simulink model "malt_test_angle"  (R2023a)
settings: Solver=FixedStepAuto  StartTime=0.0  StopTime=50  FixedStep=framePeriod_s  RelTol=1e-3
undefined symbols (not defined in the file or in its folder): Aircraft, DiscIntNeverNeededParam, framePeriod_s, frameRate_hz
libraries: simulink x29, slpidlib x8, simulink_extras x3
(part 1 of 2)
settings Model: Creator=brian  LastModifiedBy=tuan
settings SolverCC: AlgebraicLoopSolver=TrustRegion
settings OptimizationCC: DefaultParameterBehavior=Inlined  GainParamInheritBuiltInType=on  UseFloatMulNetSlope=on  DefaultUnderspecifiedDataType=single  InlineInvariantSignals=on  OptimizeBlockIOStorage=off  PassReuseOutputArgsAs=Individual arguments  ZeroExternalMemoryAtStartup=off  ZeroInternalMemoryAtStartup=off  NoFixptDivByZeroProtection=on  EfficientFloat2IntCast=on  LifeSpan=1  OptimizeBlockOrder=speed  DifferentSizesBufferReuse=on  EfficientTunableParamExpr=on
settings DebuggingCC: ParameterTunabilityLossMsg=error  UnconnectedInputMsg=warning  UnconnectedOutputMsg=warning  UnconnectedLineMsg=warning
settings HardwareCC: ProdBitPerPointer=32  ProdBitPerSizeT=32  ProdBitPerPtrDiffT=32  ProdLargestAtomicInteger=Long  ProdLargestAtomicFloat=Double  ProdWordSize=32  ProdLongLongMode=on  ProdHWDeviceType=NXP->Cortex-M4
settings ModelReferenceCC: EnableRefExpFcnMdlSchedulingChecks=on  ModelReferenceNumInstancesAllowed=Single
settings SFSimCC: SimParseCustomCode=off  MATLABDynamicMemAlloc=off  SimTargetLang=C++
settings RTWCC: Description=Embedded Coder  SystemTargetFile=ert.tlc  GenCodeOnly=on  TemplateMakefile=ert_default_tmf  GenerateReport=on  RTWVerbose=off  Toolchain=GNU gcc/g++ | gmake (64-bit Linux)  BuildConfiguration=Faster Runs  IncludeHyperlinkInReport=on  TargetLang=C++  GenerateTraceInfo=on  DLArmComputeVersion=19.05
settings CodeAppCC: ForceParamTrailComments=on  IgnoreCustomStorageClasses=off  OperatorAnnotations=on  SimulinkDataObjDesc=on  SFDataObjDesc=on  CustomSymbolStrGlobalVar=rt$N$M  CustomSymbolStrType=$N$M  CustomSymbolStrFcn=$N$M$F  CustomSymbolStrMacro=$N$M  InsertBlockDesc=on
settings ERTTargetCC: TargetLangStandard=C++11 (ISO)  IncludeMdlTerminateFcn=off  CombineSignalStateStructs=on  SuppressErrorStatus=on  SupportAbsoluteTime=off  CodeInterfacePackaging=C++ class  SupportComplex=off  ERTHeaderFileRootName=autocode$E  ERTSourceFileRootName=autocode$E  InlinedParameterPlacement=NonHierarchical  RootIOFormat=Structure reference  ERTCustomFileTemplate=example_file_process.tlc  ERTFilePackagingFormat=Compact  ArrayContainerType=std::array

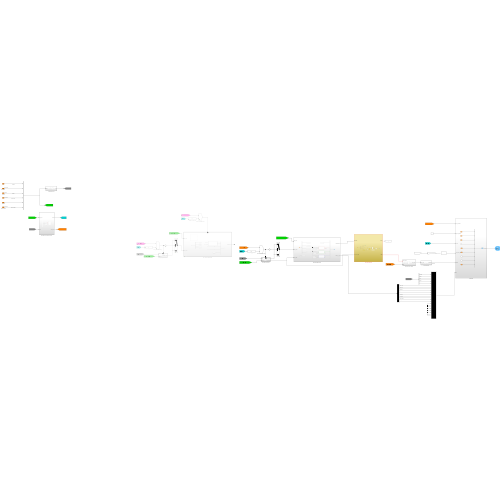
[thumbnail: Simulink's stored preview of the top-level diagram]
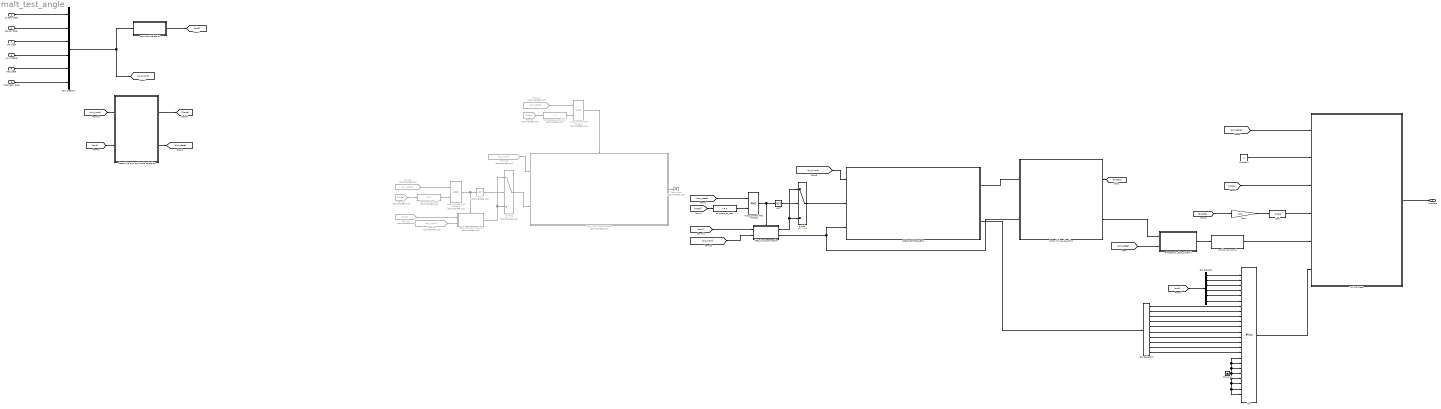
== system malt_test_angle ==
  System Data : Inport  OutDataTypeStr=Bus: SysData  SampleTime=framePeriod_s  BusOutputAsStruct=on
  Sensor Data : Inport  Port=2  OutDataTypeStr=Bus: SensorData  SampleTime=framePeriod_s  BusOutputAsStruct=on
  INS Data : Inport  Port=3  OutDataTypeStr=Bus: InsData  SampleTime=framePeriod_s  BusOutputAsStruct=on
  AuxInsData : Inport  Port=4  OutDataTypeStr=Bus: AuxInsData  SampleTime=framePeriod_s  BusOutputAsStruct=on
  ADC Data : Inport  Port=5  OutDataTypeStr=Bus: AdcData  SampleTime=framePeriod_s  BusOutputAsStruct=on
  Telemetry Data : Inport  Port=6  OutDataTypeStr=Bus: TelemData  SampleTime=framePeriod_s  BusOutputAsStruct=on
  ANGLE CONTROLLER1 : Subsystem
  Bus Creator1 : BusCreator  Inputs=6
  Bus Selector : BusSelector  OutputSignals=throttle,pitch,roll,yaw,e_stop,mode
  Bus Selector1 : BusSelector  OutputSignals=rate_cmd,rate error,signal3,signal4,signal5,D control,control cc,angle_cmd,pitch_rad,angle_e
  Cast : DataTypeConversion  OutDataTypeStr=single  SaturateOnIntegerOverflow=off  RndMeth=Floor
  Constant : Constant  Value=0  OutDataTypeStr=boolean
  From13 : From  Commented=on  GotoTag=cmd
  From15 : From  Commented=on  GotoTag=arm_state
  From16 : From  Commented=on  GotoTag=Mode
  From18 : From  Commented=on  GotoTag=sys_input
  From19 : From  Commented=on  GotoTag=sys_input
  From20 : From  Commented=on  GotoTag=arm_state
  From21 : From  Commented=on  GotoTag=Mode
  Gain : Gain  Gain=100
  Ground1 : Ground
  Motor Mixing Algorithm : Subsystem
  Mux : Mux  Inputs=24
  NOT : Logic  Operator=NOT  IconShape=distinctive  AllPortsSameDT=off  OutDataTypeStr=boolean
  NOT1 : Logic  Commented=on  Operator=NOT  IconShape=distinctive  AllPortsSameDT=off  OutDataTypeStr=boolean
  POS_HOLD CONTROLLER : Subsystem  Commented=on
  Stab_input_conversion : Subsystem
  Stab_input_conversion1 : Subsystem  Commented=on
  Switch : Switch  Criteria=u2 > Threshold  Threshold=0.5  SaturateOnIntegerOverflow=off  InputSameDT=off
  Switch1 : Switch  Commented=on  Criteria=u2 > Threshold  Threshold=0.5  SaturateOnIntegerOverflow=off  InputSameDT=off
  Terminator : Terminator  Commented=on
  To VMS Data : Subsystem
  cmd to raw pwm1 : Subsystem
  command selection : Subsystem
  compare_to_pos_hold : simulink/Logic and Bit Operations/Compare To Constant  Commented=on  relop=>  const=0  OutDataTypeStr=boolean
  compare_to_stab : simulink/Logic and Bit Operations/Compare To Constant  relop=>=  const=0  OutDataTypeStr=boolean
  compare_to_stab1 : simulink/Logic and Bit Operations/Compare To Constant  Commented=on  relop===  const=1  OutDataTypeStr=boolean
  determine arm and mode selection : Subsystem
  emergency_stop_system1 : Subsystem
  motor_armed AND mode_0 : Logic  IconShape=distinctive  AllPortsSameDT=off  OutDataTypeStr=boolean
  motor_armed AND mode_1 : Logic  Commented=on  IconShape=distinctive  AllPortsSameDT=off  OutDataTypeStr=boolean
  motor_armed AND mode_5 : Logic  Commented=on  IconShape=distinctive  AllPortsSameDT=off  OutDataTypeStr=boolean
  VmsData : Outport  OutDataTypeStr=Bus: VmsData  SampleTime=framePeriod_s  BusOutputAsStruct=on
  wires:
  To VMS Data/1(VmsData) -> VmsData/1  "VmsData"
  [Mode] -> To VMS Data/3(Mode in)
  Constant/1 -> To VMS Data/2(waypoint_reached)
  [arm_state] -> To VMS Data/1(motors_enabled)
  Cast/1 -> To VMS Data/4(throttle_cmd_prcnt)
  [throttle] -> Gain/1
  Gain/1 -> Cast/1
  determine arm and mode selection/2(arm_state) -> [arm_state]
  command selection/1(cmd) -> [cmd]
  determine arm and mode selection/1(mode) -> [Mode]
  Bus Creator1/1 -> command selection/1(InBus), [sys_input]
  [cmd] -> determine arm and mode selection/2(Cmd)
  [sys_input] -> determine arm and mode selection/1(sys_input)
  Motor Mixing Algorithm/2(PWM) -> emergency_stop_system1/1(input_signal)
  cmd to raw pwm1/1(PwmCmd) -> To VMS Data/5(PWM In)  "PwmCmd"
  emergency_stop_system1/1(pwm_cmd) -> cmd to raw pwm1/1(pwm_cmd)
  Mux/1 -> To VMS Data/6(Aux)
  [cmd] -> Bus Selector/1
  Bus Selector/1 -> Mux/1  "<throttle>"
  Bus Selector/2 -> Mux/2  "<pitch>"
  Bus Selector/3 -> Mux/3  "<roll>"
  Bus Selector/4 -> Mux/4  "<yaw>"
  Bus Selector/5 -> Mux/5  "<e_stop>"
  Bus Selector/6 -> Mux/6  "<mode>"
  [arm_state] -> emergency_stop_system1/2(arm)
  Motor Mixing Algorithm/1(throttle) -> [throttle]
  compare_to_stab/1 -> motor_armed AND mode_0/2
  [cmd] -> Stab_input_conversion/1(cmd)
  [sys_input] -> ANGLE CONTROLLER1/1(Sys_input)
  NOT/1 -> Switch/2
  [arm_state] -> motor_armed AND mode_0/1
  motor_armed AND mode_0/1 -> Stab_input_conversion/Enable, NOT/1
  Stab_input_conversion/1(angle_ctrl_input) -> Switch/3, Switch/1
  Switch/1 -> ANGLE CONTROLLER1/2(Cmd_input)
  [Mode] -> compare_to_stab/1
  ANGLE CONTROLLER1/1(Command out) -> Motor Mixing Algorithm/1(MMA Bus)
  ANGLE CONTROLLER1/2(inner_loop_log) -> Bus Selector1/1
  compare_to_pos_hold/1 -> motor_armed AND mode_1/2
  motor_armed AND mode_5/1 -> Stab_input_conversion1/Enable, NOT1/1
  From13/1 -> Stab_input_conversion1/1(cmd)
  From16/1 -> compare_to_pos_hold/1
  From15/1 -> motor_armed AND mode_1/1
  Switch1/1 -> POS_HOLD CONTROLLER/2(Cmd_input)
  NOT1/1 -> Switch1/2
  Stab_input_conversion1/1(angle_ctrl_input) -> Switch1/1, Switch1/3
  From20/1 -> motor_armed AND mode_5/1
  From19/1 -> POS_HOLD CONTROLLER/1(Sys_input)
  From21/1 -> compare_to_stab1/1
  motor_armed AND mode_1/1 -> POS_HOLD CONTROLLER/Enable
  compare_to_stab1/1 -> motor_armed AND mode_5/2
  [sys_input] -> Stab_input_conversion/2(sys input)
  Ground1/1 -> Mux/19, Mux/18, Mux/17, Mux/21, Mux/22, Mux/23, Mux/24, Mux/20
  From18/1 -> Stab_input_conversion1/2(sys input)
  Stab_input_conversion/2(low_throttle) -> ANGLE CONTROLLER1/3(low_thottle), Motor Mixing Algorithm/2(low_throttle_flag)
  System Data/1 -> Bus Creator1/1  "Sys Data"
  AuxInsData/1 -> Bus Creator1/4  "Aux Ins Data"
  Telemetry Data/1 -> Bus Creator1/6  "Telemetry Data"
  Sensor Data/1 -> Bus Creator1/2  "Sensor Data"
  INS Data/1 -> Bus Creator1/3  "Ins Data"
  ADC Data/1 -> Bus Creator1/5  "ADC Data"
  POS_HOLD CONTROLLER/1(Command out) -> Terminator/1
  Bus Selector1/2 -> Mux/8  "<rate error>"
  Bus Selector1/3 -> Mux/9  "<signal3>"
  Bus Selector1/4 -> Mux/10  "<signal4>"
  Bus Selector1/5 -> Mux/11  "<signal5>"
  Bus Selector1/6 -> Mux/12  "<D control>"
  Bus Selector1/7 -> Mux/13  "<control cc>"
  Bus Selector1/1 -> Mux/7  "<rate_cmd>"
  Bus Selector1/8 -> Mux/14  "<angle_cmd>"
  Bus Selector1/9 -> Mux/15  "<pitch_rad>"
  Bus Selector1/10 -> Mux/16  "<angle_e>"

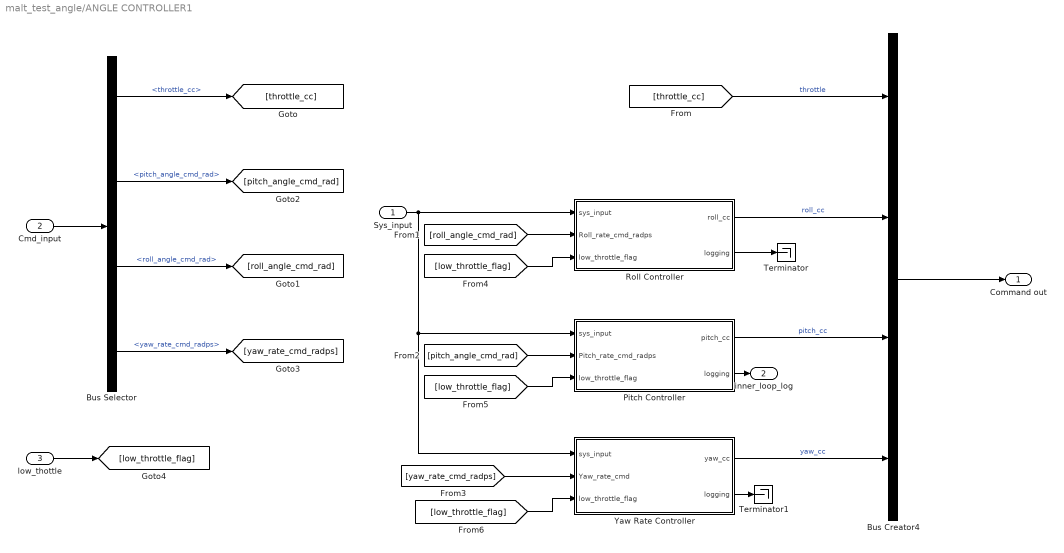
== system malt_test_angle/ANGLE CONTROLLER1 ==
  Sys_input : Inport
  Cmd_input : Inport  Port=2
  low_thottle : Inport  Port=3
  Bus Creator4 : BusCreator  Inputs=4
  Bus Selector : BusSelector  OutputSignals=throttle_cc,pitch_angle_cmd_rad,roll_angle_cmd_rad,yaw_rate_cmd_radps
  Pitch Controller : Subsystem
  Roll Controller : Subsystem
  Terminator : Terminator
  Terminator1 : Terminator
  Yaw Rate Controller : Subsystem
  Command out : Outport
  inner_loop_log : Outport  Port=2
  wires:
  Bus Creator4/1 -> Command out/1
  Cmd_input/1 -> Bus Selector/1
  Yaw Rate Controller/1(yaw_cc) -> Bus Creator4/4  "yaw_cc"
  Pitch Controller/1(pitch_cc) -> Bus Creator4/3  "pitch_cc"
  Roll Controller/1(roll_cc) -> Bus Creator4/2  "roll_cc"
  Sys_input/1 -> Yaw Rate Controller/1(sys_input), Pitch Controller/1(sys_input), Roll Controller/1(sys_input)
  Bus Selector/1 -> [throttle_cc]  "<throttle_cc>"
  Bus Selector/4 -> [yaw_rate_cmd_radps]  "<yaw_rate_cmd_radps>"
  Bus Selector/2 -> [pitch_angle_cmd_rad]  "<pitch_angle_cmd_rad>"
  Bus Selector/3 -> [roll_angle_cmd_rad]  "<roll_angle_cmd_rad>"
  [throttle_cc] -> Bus Creator4/1  "throttle"
  [roll_angle_cmd_rad] -> Roll Controller/2(Roll_rate_cmd_radps)
  [pitch_angle_cmd_rad] -> Pitch Controller/2(Pitch_rate_cmd_radps)
  [yaw_rate_cmd_radps] -> Yaw Rate Controller/2(Yaw_rate_cmd)
  low_thottle/1 -> [low_throttle_flag]
  [low_throttle_flag] -> Roll Controller/3(low_throttle_flag)
  [low_throttle_flag] -> Pitch Controller/3(low_throttle_flag)
  [low_throttle_flag] -> Yaw Rate Controller/3(low_throttle_flag)
  Roll Controller/2(logging) -> Terminator/1
  Yaw Rate Controller/2(logging) -> Terminator1/1
  Pitch Controller/2(logging) -> inner_loop_log/1

== system malt_test_angle/Motor Mixing Algorithm ==
  MMA Bus : Inport
  low_throttle_flag : Inport  Port=2
  Bus Selector : BusSelector  OutputSignals=throttle,roll_cc,pitch_cc,yaw_cc
  Constant : Constant
  Constant1 : Constant  Value=Aircraft.Control.motor_spin_min
  Constant2 : Constant  Value=[0 0 0 0 0 0 0 0]
  Motor Mix : Constant  Value=Aircraft.Motor.mix  OutDataTypeStr=single
  Multiply : Product  Inputs=**  Multiplication=Matrix(*)  OutDataTypeStr=single
  Mux : Mux
  Reshape : Reshape  OutputDimensionality=Row vector (2-D)
  Saturation Dynamic : simulink/Discontinuities/Saturation Dynamic  OutMin=[]  OutMax=[]  OutDataTypeStr=Inherit: Same as second input  OutDataType=fixdt(1, 16)  OutScaling=2^-10  DoSatur=off
  Switch : Switch  Criteria=u2 > Threshold  SaturateOnIntegerOverflow=off  InputSameDT=off
  Transpose : Math  Operator=transpose
  throttle : Outport
  PWM : Outport  Port=2
  wires:
  Mux/1 -> Reshape/1
  Reshape/1 -> Multiply/1
  Motor Mix/1 -> Transpose/1
  MMA Bus/1 -> Bus Selector/1
  Bus Selector/1 -> throttle/1, Mux/1  "<throttle>"
  Transpose/1 -> Multiply/2
  Saturation Dynamic/1 -> PWM/1
  Constant/1 -> Saturation Dynamic/1
  Constant1/1 -> Saturation Dynamic/3
  Bus Selector/2 -> Mux/2  "<roll_cc>"
  Bus Selector/3 -> Mux/3  "<pitch_cc>"
  Bus Selector/4 -> Mux/4  "<yaw_cc>"
  Switch/1 -> Saturation Dynamic/2
  low_throttle_flag/1 -> Switch/2
  Multiply/1 -> Switch/3  "Command"
  Constant2/1 -> Switch/1

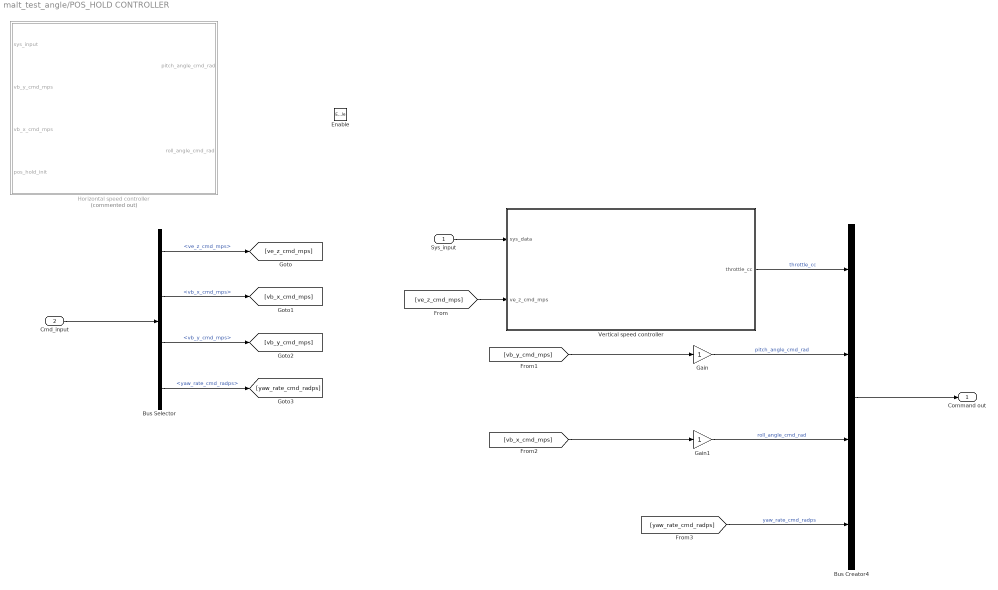
== system malt_test_angle/POS_HOLD CONTROLLER ==
  Sys_input : Inport
  Cmd_input : Inport  Port=2
  Enable : EnablePort  StatesWhenEnabling=reset  PropagateVarSize=During execution
  Bus Creator4 : BusCreator  Inputs=4
  Bus Selector : BusSelector  OutputSignals=ve_z_cmd_mps,vb_x_cmd_mps,vb_y_cmd_mps,yaw_rate_cmd_radps
  Gain : Gain
  Gain1 : Gain
  Horizontal speed controller : Subsystem  Commented=on
  Vertical speed controller : Subsystem
  Command out : Outport
  wires:
  Bus Creator4/1 -> Command out/1
  Bus Selector/1 -> [ve_z_cmd_mps]  "<ve_z_cmd_mps>"
  Bus Selector/2 -> [vb_x_cmd_mps]  "<vb_x_cmd_mps>"
  Bus Selector/3 -> [vb_y_cmd_mps]  "<vb_y_cmd_mps>"
  Bus Selector/4 -> [yaw_rate_cmd_radps]  "<yaw_rate_cmd_radps>"
  [yaw_rate_cmd_radps] -> Bus Creator4/4  "yaw_rate_cmd_radps"
  Cmd_input/1 -> Bus Selector/1
  Vertical speed controller/1(throttle_cc) -> Bus Creator4/1  "throttle_cc"
  [vb_y_cmd_mps] -> Gain/1
  [vb_x_cmd_mps] -> Gain1/1
  Sys_input/1 -> Vertical speed controller/1(sys_data)
  [ve_z_cmd_mps] -> Vertical speed controller/2(ve_z_cmd_mps)
  Gain/1 -> Bus Creator4/2  "pitch_angle_cmd_rad"
  Gain1/1 -> Bus Creator4/3  "roll_angle_cmd_rad"

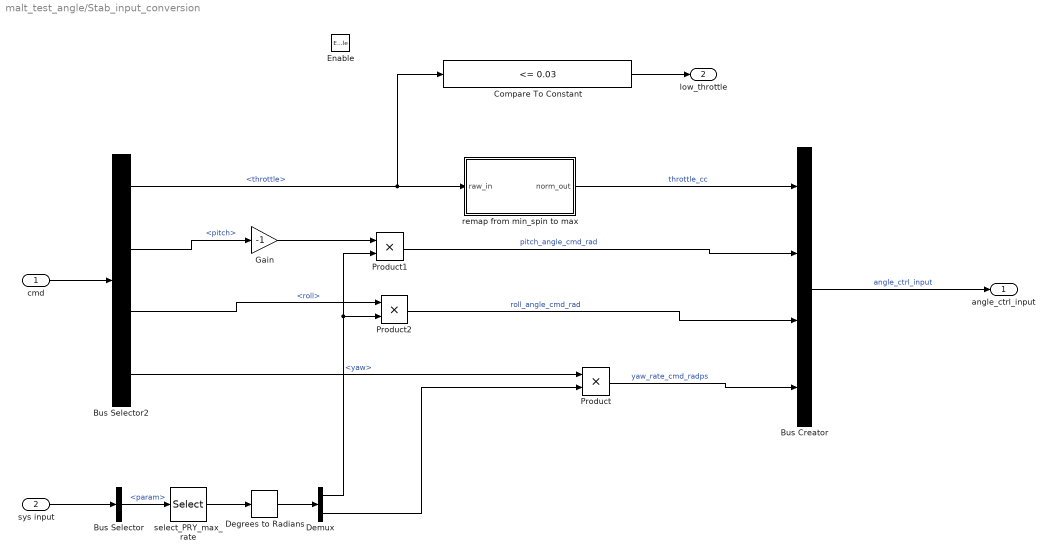
== system malt_test_angle/Stab_input_conversion ==
  cmd : Inport
  sys input : Inport  Port=2
  Enable : EnablePort
  Bus Creator : BusCreator  Inputs=4
  Bus Selector : BusSelector  OutputSignals=Telemetry Data.param
  Bus Selector2 : BusSelector  OutputSignals=throttle,pitch,roll,yaw
  Compare To Constant : simulink/Logic and Bit Operations/Compare To Constant  relop=<=  const=0.03  OutDataTypeStr=boolean
  Degrees to Radians : simulink_extras/Transformations/Degrees to Radians
  Demux : Demux  Outputs=2
  Gain : Gain  Gain=-1
  Product : Product
  Product1 : Product
  Product2 : Product
  remap from min_spin to max : Subsystem
  select_PRY_max_rate : Selector  IndexMode=Zero-based  IndexOptions=Index vector (dialog)  Indices=[13 12]  OutputSizes=1
  angle_ctrl_input : Outport
  low_throttle : Outport  Port=2
  wires:
  Bus Selector2/3 -> Product2/1  "<roll>"
  Product2/1 -> Bus Creator/3  "roll_angle_cmd_rad"
  Bus Selector2/2 -> Gain/1  "<pitch>"
  Bus Creator/1 -> angle_ctrl_input/1  "angle_ctrl_input"
  Product1/1 -> Bus Creator/2  "pitch_angle_cmd_rad"
  cmd/1 -> Bus Selector2/1
  Bus Selector2/1 -> Compare To Constant/1, remap from min_spin to max/1(raw_in)  "<throttle>"
  Product/1 -> Bus Creator/4  "yaw_rate_cmd_radps"
  Bus Selector2/4 -> Product/1  "<yaw>"
  remap from min_spin to max/1(norm_out) -> Bus Creator/1  "throttle_cc"
  Compare To Constant/1 -> low_throttle/1
  sys input/1 -> Bus Selector/1
  Bus Selector/1 -> select_PRY_max_rate/1  "<param>"
  select_PRY_max_rate/1 -> Degrees to Radians/1
  Demux/2 -> Product/2
  Gain/1 -> Product1/1
  Demux/1 -> Product2/2, Product1/2
  Degrees to Radians/1 -> Demux/1

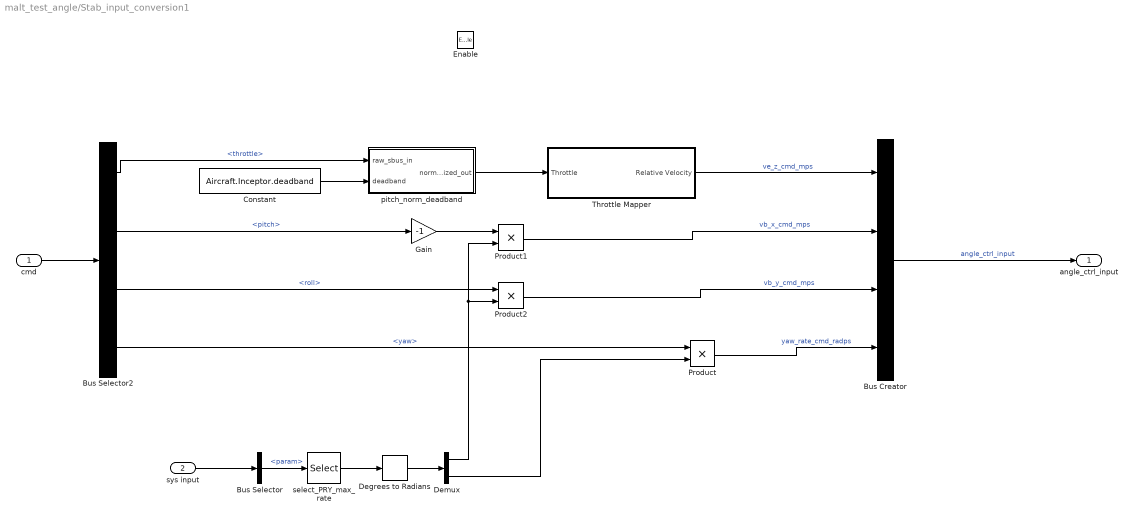
== system malt_test_angle/Stab_input_conversion1 ==
  cmd : Inport
  sys input : Inport  Port=2
  Enable : EnablePort
  Bus Creator : BusCreator  Inputs=4
  Bus Selector : BusSelector  OutputSignals=Telemetry Data.param
  Bus Selector2 : BusSelector  OutputSignals=throttle,pitch,roll,yaw
  Constant : Constant  Value=Aircraft.Inceptor.deadband
  Degrees to Radians : simulink_extras/Transformations/Degrees to Radians
  Demux : Demux  Outputs=2
  Gain : Gain  Gain=-1
  Product : Product
  Product1 : Product
  Product2 : Product
  Throttle Mapper : Subsystem
  pitch_norm_deadband : Subsystem
  select_PRY_max_rate : Selector  IndexMode=Zero-based  IndexOptions=Index vector (dialog)  Indices=[13 12]  OutputSizes=1
  angle_ctrl_input : Outport
  wires:
  Bus Selector2/3 -> Product2/1  "<roll>"
  Product2/1 -> Bus Creator/3  "vb_y_cmd_mps"
  Bus Selector2/2 -> Gain/1  "<pitch>"
  Bus Creator/1 -> angle_ctrl_input/1  "angle_ctrl_input"
  Product1/1 -> Bus Creator/2  "vb_x_cmd_mps"
  cmd/1 -> Bus Selector2/1
  Product/1 -> Bus Creator/4  "yaw_rate_cmd_radps"
  Bus Selector2/4 -> Product/1  "<yaw>"
  Throttle Mapper/1(Relative Velocity) -> Bus Creator/1  "ve_z_cmd_mps"
  sys input/1 -> Bus Selector/1
  Bus Selector/1 -> select_PRY_max_rate/1  "<param>"
  select_PRY_max_rate/1 -> Degrees to Radians/1
  Demux/2 -> Product/2
  Gain/1 -> Product1/1
  Demux/1 -> Product2/2, Product1/2
  Degrees to Radians/1 -> Demux/1
  Bus Selector2/1 -> pitch_norm_deadband/1(raw_sbus_in)  "<throttle>"
  pitch_norm_deadband/1(normalized_out) -> Throttle Mapper/1(Throttle)
  Constant/1 -> pitch_norm_deadband/2(deadband)

== system malt_test_angle/To VMS Data ==
  motors_enabled : Inport
  waypoint_reached : Inport  Port=2
  Mode in : Inport  Port=3
  throttle_cmd_prcnt : Inport  Port=4
  PWM In : Inport  Port=5
  Aux : Inport  Port=6
  Bus Creator : BusCreator  Inputs=9  OutDataTypeStr=Bus: VmsData  NonVirtualBus=on
      settings: InheritFromInputs=off
  Ground : Ground
  Ground1 : Ground
  Ground2 : Ground
  VmsData : Outport
  wires:
  Bus Creator/1 -> VmsData/1
  waypoint_reached/1 -> Bus Creator/1  "advance_waypoint"
  motors_enabled/1 -> Bus Creator/2  "motors_enabled"
  Mode in/1 -> Bus Creator/3  "mode"
  Ground1/1 -> Bus Creator/4  "sbus"
  PWM In/1 -> Bus Creator/5  "pwm"
  throttle_cmd_prcnt/1 -> Bus Creator/6  "throttle_cmd_prcnt"
  Aux/1 -> Bus Creator/9  "aux"
  Ground/1 -> Bus Creator/7  "flight_time_remaining_s"
  Ground2/1 -> Bus Creator/8  "power_remaining_prcnt"

== system malt_test_angle/cmd to raw pwm1 ==
  note: cnt - pwm output to actual hardware
  pwm_cmd : Inport
  Data Type Conversion : DataTypeConversion  OutDataTypeStr=int16  SaturateOnIntegerOverflow=off  RndMeth=Floor
  motor_PWM_denormalize : Subsystem
  PwmCmd : Outport
  wires:
  pwm_cmd/1 -> motor_PWM_denormalize/1(normalized_input)  "cmd"
  motor_PWM_denormalize/1(raw_output) -> Data Type Conversion/1
  Data Type Conversion/1 -> PwmCmd/1  "cnt"

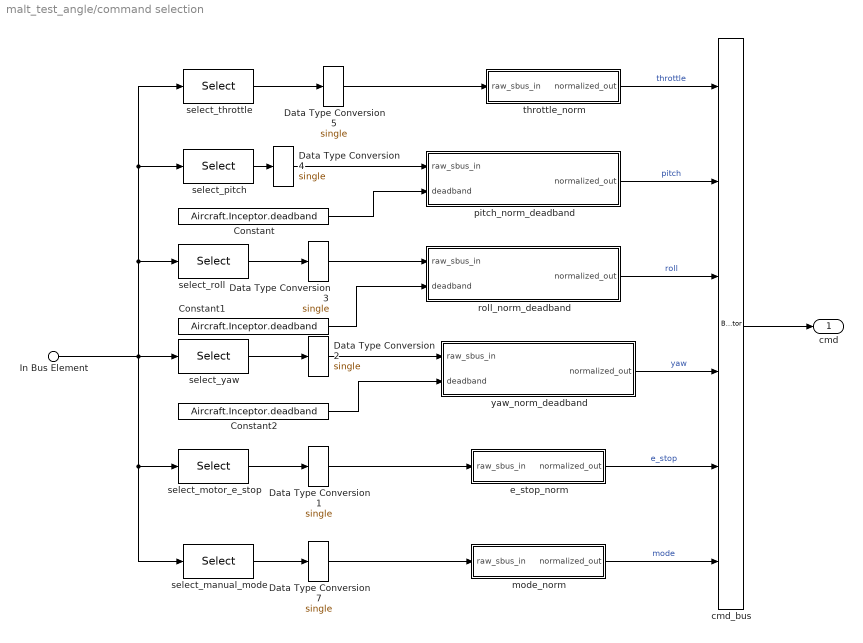
== system malt_test_angle/command selection ==
  In Bus Element : Inport  PortName=InBus  Element=Sensor Data.inceptor.ch
  Constant : Constant  Value=Aircraft.Inceptor.deadband
  Constant1 : Constant  Value=Aircraft.Inceptor.deadband
  Constant2 : Constant  Value=Aircraft.Inceptor.deadband
  Data Type Conversion{1..5,7} (6 alike) : DataTypeConversion  OutDataTypeStr=single  SaturateOnIntegerOverflow=off  RndMeth=Floor
  cmd_bus : BusCreator  Inputs=6
  e_stop_norm : Subsystem
  mode_norm : Subsystem
  pitch_norm_deadband : Subsystem
  roll_norm_deadband : Subsystem
  select_manual_mode : Selector  IndexOptions=Index vector (dialog)  Indices=Aircraft.Inceptor.mode0  OutputSizes=1
  select_motor_e_stop : Selector  IndexOptions=Index vector (dialog)  Indices=Aircraft.Inceptor.throttle_e_stop  OutputSizes=1
  select_pitch : Selector  IndexOptions=Index vector (dialog)  Indices=Aircraft.Inceptor.pitch  OutputSizes=1
  select_roll : Selector  IndexOptions=Index vector (dialog)  Indices=Aircraft.Inceptor.roll  OutputSizes=1
  select_throttle : Selector  IndexOptions=Index vector (dialog)  Indices=Aircraft.Inceptor.throttle  OutputSizes=1
  select_yaw : Selector  IndexOptions=Index vector (dialog)  Indices=Aircraft.Inceptor.yaw  OutputSizes=1
  throttle_norm : Subsystem
  yaw_norm_deadband : Subsystem
  cmd : Outport
  wires:
  select_pitch/1 -> Data Type Conversion4/1
  select_yaw/1 -> Data Type Conversion2/1
  select_throttle/1 -> Data Type Conversion5/1
  cmd_bus/1 -> cmd/1
  Data Type Conversion5/1 -> throttle_norm/1(raw_sbus_in)
  select_roll/1 -> Data Type Conversion3/1
  In Bus Element/1 -> select_roll/1, select_throttle/1, select_pitch/1, select_manual_mode/1, select_motor_e_stop/1, select_yaw/1
  Data Type Conversion1/1 -> e_stop_norm/1(raw_sbus_in)
  select_motor_e_stop/1 -> Data Type Conversion1/1
  Data Type Conversion7/1 -> mode_norm/1(raw_sbus_in)
  select_manual_mode/1 -> Data Type Conversion7/1
  Data Type Conversion2/1 -> yaw_norm_deadband/1(raw_sbus_in)
  Constant2/1 -> yaw_norm_deadband/2(deadband)
  throttle_norm/1(normalized_out) -> cmd_bus/1  "throttle"
  roll_norm_deadband/1(normalized_out) -> cmd_bus/3  "roll"
  pitch_norm_deadband/1(normalized_out) -> cmd_bus/2  "pitch"
  Data Type Conversion4/1 -> pitch_norm_deadband/1(raw_sbus_in)
  Constant/1 -> pitch_norm_deadband/2(deadband)
  Constant1/1 -> roll_norm_deadband/2(deadband)
  Data Type Conversion3/1 -> roll_norm_deadband/1(raw_sbus_in)
  yaw_norm_deadband/1(normalized_out) -> cmd_bus/4  "yaw"
  e_stop_norm/1(normalized_out) -> cmd_bus/5  "e_stop"
  mode_norm/1(normalized_out) -> cmd_bus/6  "mode"

== system malt_test_angle/determine arm and mode selection ==
  sys_input : Inport
  Cmd : Inport  Port=2
  Bus Selector : BusSelector  OutputSignals=Sensor Data.inceptor,Ins Data.initialized
  Bus Selector1 : BusSelector  OutputSignals=e_stop,mode,yaw,throttle
  Failsafe_management : Subsystem
  OR1 : Logic  Operator=OR  IconShape=distinctive  AllPortsSameDT=off  OutDataTypeStr=boolean
  Subsystem : Subsystem
  mode_type_conversion : DataTypeConversion  OutDataTypeStr=int8  RndMeth=Nearest  SaturateOnIntegerOverflow=off
  nav_init AND motor_enable : Logic  IconShape=distinctive  AllPortsSameDT=off  OutDataTypeStr=boolean
  yaw_stick_arming : Subsystem
  mode : Outport
  arm_state : Outport  Port=2
  wires:
  Failsafe_management/1(radio_failsafe_enabled) -> [radio_failsafe_enabled]
  nav_init AND motor_enable/1 -> arm_state/1, Failsafe_management/3(motor_state)
  Bus Selector/2 -> nav_init AND motor_enable/2  "<initialized>"
  sys_input/1 -> Bus Selector/1
  [motor_e_stop] -> yaw_stick_arming/3(e_stop)
  Bus Selector1/4 -> yaw_stick_arming/2(<throttle>)  "<throttle>"
  Bus Selector1/2 -> mode_type_conversion/1  "<mode>"
  Bus Selector1/3 -> yaw_stick_arming/1(<yaw>)  "<yaw>"
  Bus Selector1/1 -> Subsystem/1(<e_stop>)  "<e_stop>"
  mode_type_conversion/1 -> mode/1, Failsafe_management/2(manual_mode)
  Cmd/1 -> Bus Selector1/1
  yaw_stick_arming/1(arm_state) -> nav_init AND motor_enable/1
  OR1/1 -> [motor_e_stop]
  [radio_failsafe_enabled] -> OR1/2
  Subsystem/1(e_stop_filtered) -> OR1/1
  Bus Selector/1 -> Failsafe_management/1(failsafe)  "<inceptor>"

== system malt_test_angle/emergency_stop_system1 ==
  input_signal : Inport
  arm : Inport  Port=2
  Constant : Constant  Value=[0,0,0,0,0,0,0,0]  OutDataTypeStr=single
  emergency_switch : Switch  Criteria=u2 > Threshold  Threshold=0.5  SaturateOnIntegerOverflow=off  InputSameDT=off
  pwm_cmd : Outport
  wires:
  emergency_switch/1 -> pwm_cmd/1
  arm/1 -> emergency_switch/2
  input_signal/1 -> emergency_switch/1
  Constant/1 -> emergency_switch/3

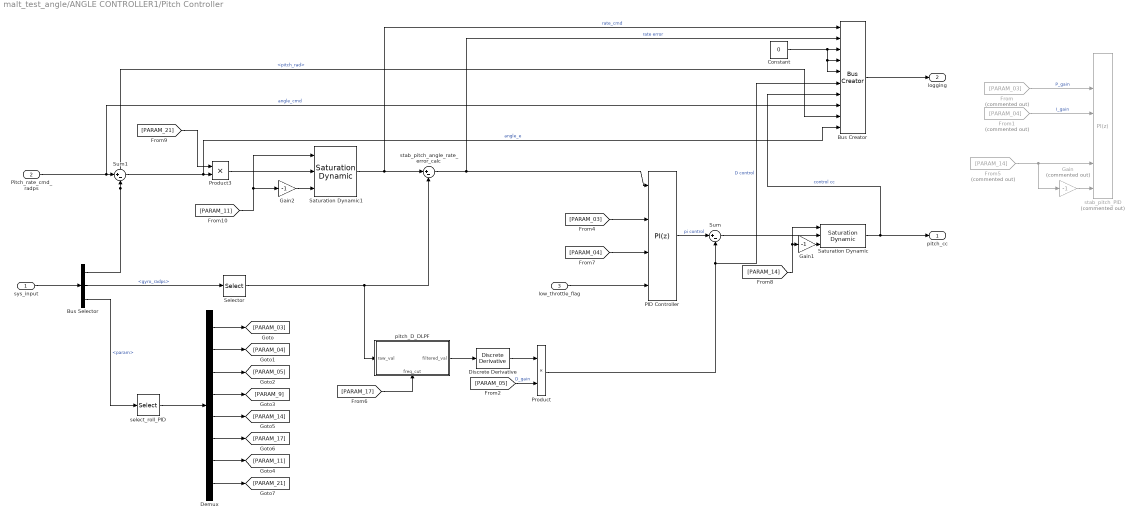
== system malt_test_angle/ANGLE CONTROLLER1/Pitch Controller ==
  sys_input : Inport
  Pitch_rate_cmd_radps : Inport  Port=2
  low_throttle_flag : Inport  Port=3
  Bus Creator : BusCreator  Inputs=10
  Bus Selector : BusSelector  OutputSignals=Ins Data.pitch_rad,Ins Data.gyro_radps,Telemetry Data.param
  Constant : Constant  Value=0  OutDataTypeStr=single
  Demux : Demux  Outputs=8
  Discrete Derivative : simulink/Discrete/Discrete Derivative  gainval=1.0  ICPrevScaledInput=0.0  OutMin=[]  OutMax=[]  OutDataType=fixdt(1, 16)  OutScaling=2^-10  DoSatur=off
  From : From  Commented=on  GotoTag=PARAM_03
  From1 : From  Commented=on  GotoTag=PARAM_04
  From5 : From  Commented=on  GotoTag=PARAM_14
  Gain : Gain  Commented=on  Gain=-1
  Gain1 : Gain  Gain=-1
  Gain2 : Gain  Gain=-1
  PID Controller : slpidlib/PID Controller  Controller=PI  Form=Parallel  TimeDomain=Discrete-time  UseExternalTs=off  SampleTime=framePeriod_s  IntegratorMethod=Forward Euler  FilterMethod=Forward Euler  ControllerParametersSource=external  P=1  I=1  UseKiTs=off  D=0  N=100  UseFilter=on  TunerSelectOption=Transfer Function Based (PID Tuner App)  InitialConditionSource=internal  InitialConditionForIntegrator=0  InitialConditionForFilter=0  DifferentiatorICPrevScaledInput=0  ExternalReset=either  TrackingMode=off  Kt=1  LimitOutput=on  SatLimitsSource=internal  UpperSaturationLimit=1  LowerSaturationLimit=-1  LinearizeAsGain=on  AntiWindupMode=clamping  Kb=1  LimitIntegrator=off  UpperIntegratorSaturationLimit=inf  LowerIntegratorSaturationLimit=-inf  POutMin=[]  POutMax=[]  IOutMin=[]  IOutMax=[]  DOutMin=[]  DOutMax=[]  NOutMin=[]  NOutMax=[]  SumOutMin=[]  SumOutMax=[]  SaturationOutMin=[]  SaturationOutMax=[]  PParamMin=[]  PParamMax=[]  IParamMin=[]  IParamMax=[]  DParamMin=[]  DParamMax=[]  NParamMin=[]  NParamMax=[]  KbParamMin=[]  KbParamMax=[]  KtParamMin=[]  KtParamMax=[]  KbOutMin=[]  KbOutMax=[]  KtOutMin=[]  KtOutMax=[]  IntegratorOutMin=[]  IntegratorOutMax=[]  FilterOutMin=[]  FilterOutMax=[]  SumI1OutMin=[]  SumI1OutMax=[]  SumI2OutMin=[]  SumI2OutMax=[]  SumI3OutMin=[]  SumI3OutMax=[]  SumI4OutMin=[]  SumI4OutMax=[]  SumDOutMin=[]  SumDOutMax=[]  DifferentiatorOutMin=[]  DifferentiatorOutMax=[]  FilterDiffOutCoefMin=[]  FilterDiffOutCoefMax=[]  ReciprocalOutMin=[]  ReciprocalOutMax=[]  SumDenOutMin=[]  SumDenOutMax=[]  SumNumOutMin=[]  SumNumOutMax=[]  DivideOutMin=[]  DivideOutMax=[]  UdiffTsProdOutMin=[]  UdiffTsProdOutMax=[]  NTsProdOutMin=[]  NTsProdOutMax=[]  UintegralTsProdOutMin=[]  UintegralTsProdOutMax=[]  UngainTsProdOutMin=[]  UngainTsProdOutMax=[]  ClampingZeroOutDataTypeStr=Inherit: Inherit via back propagation  ClampingZeroOutMin=[]  ClampingZeroOutMax=[]  FilterDenConstantOutDataTypeStr=Inherit: Inherit via back propagation  FilterDenConstantOutMin=[]  FilterDenConstantOutMax=[]  PCopyOutDataTypeStr=Inherit: Inherit via back propagation  PCopyOutMin=[]  PCopyOutMax=[]  NCopyOutDataTypeStr=Inherit: Inherit via back propagation  NCopyOutMin=[]  NCopyOutMax=[]  IntegratorContinuousStateAttributes=''  IntegratorStateMustResolveToSignalObject=off  IntegratorRTWStateStorageClass=Auto  FilterContinuousStateAttributes=''  FilterStateMustResolveToSignalObject=off  FilterRTWStateStorageClass=Auto  ParallelPVariant=ExternalParameters  IdealPVariant=Disabled  IVariant=ExternalParameters  DVariant=Disabled  IntegratorVariant=Discrete  SatVariant=Enabled  AWVariant=DiscClampingParallel  PCopyVariant=Disabled  TRVariant=Disabled  FdbkBlocksVariant=Forward  IdealPFdbkVariant=Disabled  SatFdbkVariant=Disabled  DerivativeFilterVariant=Disabled  NVariant=Disabled  NCopyVariant=Disabled_SignalSpec  FilterICVariant=Disabled  IntegratorICVariant=InternalICs  ExternalResetVariant=ExternalReset  TRSumVariant=Passthrough  SumFdbkVariant=Disabled  SumVariant=Sum_PI  TsampFilterVariant=InternalTs  TsampNgainVariant=Passthrough  TsampIntegralVariant=Disabled_SignalSpec  ExternalSaturationOutDataTypeStr=Inherit: Same as second input
  Product : Product
  Product3 : Product
  Saturation Dynamic : simulink/Discontinuities/Saturation Dynamic  OutMin=[]  OutMax=[]  OutDataTypeStr=Inherit: Same as second input  OutDataType=fixdt(1, 16)  OutScaling=2^-10  DoSatur=off
  Saturation Dynamic1 : simulink/Discontinuities/Saturation Dynamic  OutMin=[]  OutMax=[]  OutDataTypeStr=Inherit: Same as second input  OutDataType=fixdt(1, 16)  OutScaling=2^-10  DoSatur=off
  Selector : Selector  IndexMode=Zero-based  InputPortWidth=3  IndexOptions=Index vector (dialog)  Indices=1  OutputSizes=1
  Sum : Sum  Inputs=|+-
  Sum1 : Sum  Inputs=|+-
  pitch_D_DLPF : Subsystem
      settings: PortSchema="{\"entries\":[{\"content\":{\"sides\":[{\"content\":{\"connectorIds\":[\"In1\"]},\"type\":\"ConnectorPlacement.EquallySpacedRectSide\",\"uuid\":\"20236834-aeb3-4c5b-bb2e-f84447e752b5\"},{\"content\":{\"connectorIds\":[\"Out1\"],\"side\":\"RIGHT\"},\"type\":\"ConnectorPlacement.EquallySpacedRectSide\",\"uuid\":\"d668f9a1-a3df-4207-8bf1-99fb838e59b2\"},{\"content\":{\"connectorIds\":[],\"side\":\"TOP\"},\"type\":\"ConnectorPlacement.EquallySpacedRectSide\",\"uuid\":\"66cceb06-f4bc-4278-b965-2427292e46df\"},{\"content\":{\"connectorIds\":[\"In2\"],\"side\":\"BOTTOM\"},\"type\":\"ConnectorPlacement.EquallySpacedRectSide\",\"uuid\":\"8fdaac6a-cb03-4bd4-87bb-7bafd10bc297\"}]},\"type\":\"ConnectorPlacement.EquallySpacedConnector\",\"uuid\":\"3dc29a9a-e794-478d-b7df-452e6c2d3f66\"}],\"packageUris\":[\"http://schema.mathworks.com/mf0/Connector/R2020b\"],\"version\":\"1.0\"}"
  select_roll_PID : Selector  IndexMode=Zero-based  IndexOptions=Index vector (dialog)  Indices=[3 4 5 9 14 17 11 21]  OutputSizes=1
  stab_pitch_PID : slpidlib/PID Controller  Commented=on  Controller=PI  Form=Parallel  TimeDomain=Discrete-time  UseExternalTs=off  SampleTime=framePeriod_s  IntegratorMethod=Forward Euler  FilterMethod=Forward Euler  ControllerParametersSource=external  P=0.335  I=0.005  UseKiTs=off  D=0  N=100  UseFilter=off  TunerSelectOption=Transfer Function Based (PID Tuner App)  InitialConditionSource=internal  InitialConditionForIntegrator=0  InitialConditionForFilter=0  DifferentiatorICPrevScaledInput=0  ExternalReset=either  TrackingMode=off  Kt=1  LimitOutput=on  SatLimitsSource=external  UpperSaturationLimit=inf  LowerSaturationLimit=-inf  LinearizeAsGain=on  AntiWindupMode=clamping  Kb=1  LimitIntegrator=off  UpperIntegratorSaturationLimit=inf  LowerIntegratorSaturationLimit=-inf  POutMin=[]  POutMax=[]  IOutMin=[]  IOutMax=[]  DOutMin=[]  DOutMax=[]  NOutMin=[]  NOutMax=[]  SumOutMin=[]  SumOutMax=[]  SaturationOutMin=[]  SaturationOutMax=[]  PParamMin=[]  PParamMax=[]  IParamMin=[]  IParamMax=[]  DParamMin=[]  DParamMax=[]  NParamMin=[]  NParamMax=[]  KbParamMin=[]  KbParamMax=[]  KtParamMin=[]  KtParamMax=[]  KbOutMin=[]  KbOutMax=[]  KtOutMin=[]  KtOutMax=[]  IntegratorOutMin=[]  IntegratorOutMax=[]  FilterOutMin=[]  FilterOutMax=[]  SumI1OutMin=[]  SumI1OutMax=[]  SumI2OutMin=[]  SumI2OutMax=[]  SumI3OutMin=[]  SumI3OutMax=[]  SumI4OutMin=[]  SumI4OutMax=[]  SumDOutMin=[]  SumDOutMax=[]  DifferentiatorOutMin=[]  DifferentiatorOutMax=[]  FilterDiffOutCoefMin=[]  FilterDiffOutCoefMax=[]  ReciprocalOutMin=[]  ReciprocalOutMax=[]  SumDenOutMin=[]  SumDenOutMax=[]  SumNumOutMin=[]  SumNumOutMax=[]  DivideOutMin=[]  DivideOutMax=[]  UdiffTsProdOutMin=[]  UdiffTsProdOutMax=[]  NTsProdOutMin=[]  NTsProdOutMax=[]  UintegralTsProdOutMin=[]  UintegralTsProdOutMax=[]  UngainTsProdOutMin=[]  UngainTsProdOutMax=[]  ClampingZeroOutDataTypeStr=Inherit: Inherit via back propagation  ClampingZeroOutMin=[]  ClampingZeroOutMax=[]  FilterDenConstantOutDataTypeStr=Inherit: Inherit via back propagation  FilterDenConstantOutMin=[]  FilterDenConstantOutMax=[]  PCopyOutDataTypeStr=Inherit: Inherit via back propagation  PCopyOutMin=[]  PCopyOutMax=[]  NCopyOutDataTypeStr=Inherit: Inherit via back propagation  NCopyOutMin=[]  NCopyOutMax=[]  IntegratorContinuousStateAttributes=''  IntegratorStateMustResolveToSignalObject=off  IntegratorRTWStateStorageClass=Auto  FilterContinuousStateAttributes=''  FilterStateMustResolveToSignalObject=off  FilterRTWStateStorageClass=Auto  ParallelPVariant=ExternalParameters  IdealPVariant=Disabled  IVariant=ExternalParameters  DVariant=Disabled  IntegratorVariant=Discrete  SatVariant=External  AWVariant=DiscClampingParallel  PCopyVariant=Disabled  TRVariant=Disabled  FdbkBlocksVariant=Forward  IdealPFdbkVariant=Disabled  SatFdbkVariant=Disabled  DerivativeFilterVariant=Disabled  NVariant=Disabled  NCopyVariant=Disabled_SignalSpec  FilterICVariant=Disabled  IntegratorICVariant=InternalICs  ExternalResetVariant=ExternalReset  TRSumVariant=Passthrough  SumFdbkVariant=Disabled  SumVariant=Sum_PI  TsampFilterVariant=InternalTs  TsampNgainVariant=Passthrough  TsampIntegralVariant=Disabled_SignalSpec  ExternalSaturationOutDataTypeStr=Inherit: Same as second input
  stab_pitch_angle_rate_error_calc : Sum  Inputs=|+-
  pitch_cc : Outport
  logging : Outport  Port=2
  wires:
  sys_input/1 -> Bus Selector/1
  Sum/1 -> Saturation Dynamic/2
  Bus Creator/1 -> logging/1
  Bus Selector/2 -> Selector/1  "<gyro_radps>"
  Bus Selector/3 -> select_roll_PID/1  "<param>"
  From/1 -> stab_pitch_PID/2  "P_gain"
  From1/1 -> stab_pitch_PID/3  "I_gain"
  [PARAM_05] -> Product/2  "D_gain"
  From5/1 -> Gain/1, stab_pitch_PID/5
  Gain/1 -> stab_pitch_PID/6
  Selector/1 -> pitch_D_DLPF/1(raw_val), stab_pitch_angle_rate_error_calc/2
  Discrete Derivative/1 -> Product/1
  select_roll_PID/1 -> Demux/1
  Demux/2 -> [PARAM_04]
  Demux/3 -> [PARAM_05]
  Demux/4 -> [PARAM_9]
  Demux/1 -> [PARAM_03]
  Demux/6 -> [PARAM_17]
  Demux/5 -> [PARAM_14]
  [PARAM_17] -> pitch_D_DLPF/2(freq_cut)
  pitch_D_DLPF/1(filtered_val) -> Discrete Derivative/1
  Product/1 -> Sum/2, Bus Creator/6  "D control"
  stab_pitch_angle_rate_error_calc/1 -> PID Controller/1, Bus Creator/2  "rate error"
  [PARAM_03] -> PID Controller/2
  low_throttle_flag/1 -> PID Controller/4
  [PARAM_04] -> PID Controller/3
  Saturation Dynamic/1 -> Bus Creator/7, pitch_cc/1  "control cc"
  [PARAM_14] -> Gain1/1, Saturation Dynamic/1
  Gain1/1 -> Saturation Dynamic/3
  Bus Selector/1 -> Sum1/2, Bus Creator/9  "<pitch_rad>"
  Pitch_rate_cmd_radps/1 -> Bus Creator/8, Sum1/1  "angle_cmd"
  Sum1/1 -> Bus Creator/10, Product3/2  "angle_e"
  Demux/7 -> [PARAM_11]
  Demux/8 -> [PARAM_21]
  [PARAM_21] -> Product3/1
  Product3/1 -> Saturation Dynamic1/2
  Saturation Dynamic1/1 -> Bus Creator/1, stab_pitch_angle_rate_error_calc/1  "rate_cmd"
  [PARAM_11] -> Saturation Dynamic1/1, Gain2/1
  Gain2/1 -> Saturation Dynamic1/3
  Constant/1 -> Bus Creator/5, Bus Creator/4, Bus Creator/3
  PID Controller/1 -> Sum/1  "pi control"

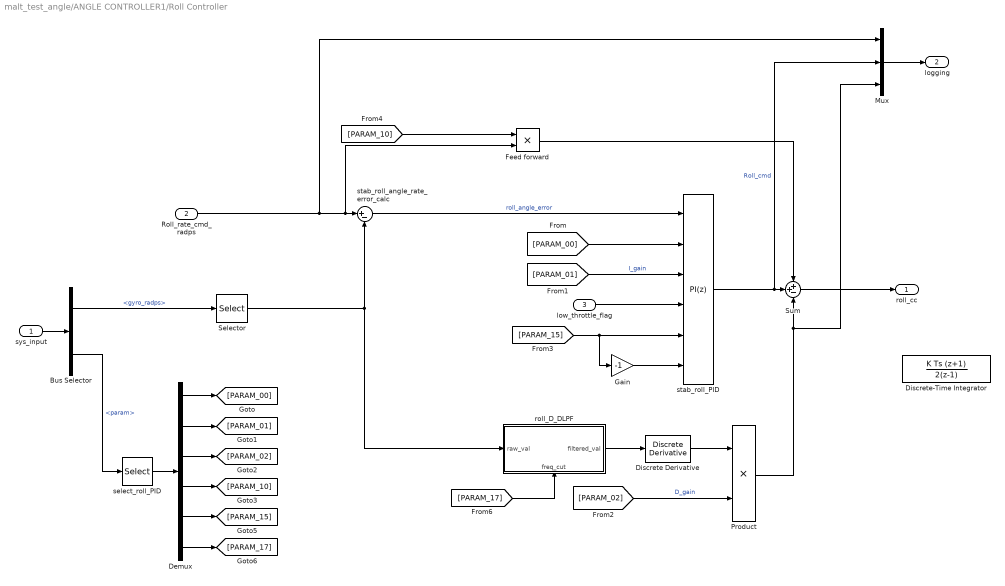
== system malt_test_angle/ANGLE CONTROLLER1/Roll Controller ==
  sys_input : Inport
  Roll_rate_cmd_radps : Inport  Port=2
  low_throttle_flag : Inport  Port=3
  Bus Selector : BusSelector  OutputSignals=Ins Data.gyro_radps,Telemetry Data.param
  Demux : Demux  Outputs=6
  Discrete Derivative : simulink/Discrete/Discrete Derivative  gainval=1.0  ICPrevScaledInput=0.0  OutMin=[]  OutMax=[]  OutDataType=fixdt(1, 16)  OutScaling=2^-10  DoSatur=off
  Discrete-Time Integrator : DiscreteIntegrator  IntegratorMethod=Integration: Trapezoidal  ExternalReset=either  SampleTime=-1  LimitOutput=on  ShowSaturationPort=on  ShowStatePort=on  ICPrevOutput=DiscIntNeverNeededParam  ICPrevScaledInput=DiscIntNeverNeededParam
  Feed forward : Product
  Gain : Gain  Gain=-1
  Mux : Mux  Inputs=3
  Product : Product
  Selector : Selector  IndexMode=Zero-based  InputPortWidth=3  IndexOptions=Index vector (dialog)  Indices=0  OutputSizes=1
  Sum : Sum  Inputs=++-
  roll_D_DLPF : Subsystem
      settings: PortSchema="{\"entries\":[{\"content\":{\"sides\":[{\"content\":{\"connectorIds\":[\"In1\"]},\"type\":\"ConnectorPlacement.EquallySpacedRectSide\",\"uuid\":\"20236834-aeb3-4c5b-bb2e-f84447e752b5\"},{\"content\":{\"connectorIds\":[\"Out1\"],\"side\":\"RIGHT\"},\"type\":\"ConnectorPlacement.EquallySpacedRectSide\",\"uuid\":\"d668f9a1-a3df-4207-8bf1-99fb838e59b2\"},{\"content\":{\"connectorIds\":[],\"side\":\"TOP\"},\"type\":\"ConnectorPlacement.EquallySpacedRectSide\",\"uuid\":\"66cceb06-f4bc-4278-b965-2427292e46df\"},{\"content\":{\"connectorIds\":[\"In2\"],\"side\":\"BOTTOM\"},\"type\":\"ConnectorPlacement.EquallySpacedRectSide\",\"uuid\":\"8fdaac6a-cb03-4bd4-87bb-7bafd10bc297\"}]},\"type\":\"ConnectorPlacement.EquallySpacedConnector\",\"uuid\":\"3dc29a9a-e794-478d-b7df-452e6c2d3f66\"}],\"packageUris\":[\"http://schema.mathworks.com/mf0/Connector/R2020b\"],\"version\":\"1.0\"}"
  select_roll_PID : Selector  IndexMode=Zero-based  IndexOptions=Index vector (dialog)  Indices=[0 1 2 10 15 17]  OutputSizes=1
  stab_roll_PID : slpidlib/PID Controller  Controller=PI  Form=Parallel  TimeDomain=Discrete-time  UseExternalTs=off  SampleTime=framePeriod_s  IntegratorMethod=Forward Euler  FilterMethod=Forward Euler  ControllerParametersSource=external  P=0.335  I=0.005  UseKiTs=off  D=0  N=100  UseFilter=off  TunerSelectOption=Transfer Function Based (PID Tuner App)  InitialConditionSource=internal  InitialConditionForIntegrator=0  InitialConditionForFilter=0  DifferentiatorICPrevScaledInput=0  ExternalReset=either  TrackingMode=off  Kt=1  LimitOutput=on  SatLimitsSource=external  UpperSaturationLimit=inf  LowerSaturationLimit=-inf  LinearizeAsGain=on  AntiWindupMode=clamping  Kb=1  POutMin=[]  POutMax=[]  IOutMin=[]  IOutMax=[]  DOutMin=[]  DOutMax=[]  NOutMin=[]  NOutMax=[]  SumOutMin=[]  SumOutMax=[]  SaturationOutMin=[]  SaturationOutMax=[]  PParamMin=[]  PParamMax=[]  IParamMin=[]  IParamMax=[]  DParamMin=[]  DParamMax=[]  NParamMin=[]  NParamMax=[]  KbParamMin=[]  KbParamMax=[]  KtParamMin=[]  KtParamMax=[]  KbOutMin=[]  KbOutMax=[]  KtOutMin=[]  KtOutMax=[]  IntegratorOutMin=[]  IntegratorOutMax=[]  FilterOutMin=[]  FilterOutMax=[]  SumI1OutMin=[]  SumI1OutMax=[]  SumI2OutMin=[]  SumI2OutMax=[]  SumI3OutMin=[]  SumI3OutMax=[]  SumI4OutMin=[]  SumI4OutMax=[]  SumDOutMin=[]  SumDOutMax=[]  DifferentiatorOutMin=[]  DifferentiatorOutMax=[]  FilterDiffOutCoefMin=[]  FilterDiffOutCoefMax=[]  ReciprocalOutMin=[]  ReciprocalOutMax=[]  SumDenOutMin=[]  SumDenOutMax=[]  SumNumOutMin=[]  SumNumOutMax=[]  DivideOutMin=[]  DivideOutMax=[]  UdiffTsProdOutMin=[]  UdiffTsProdOutMax=[]  NTsProdOutMin=[]  NTsProdOutMax=[]  UintegralTsProdOutMin=[]  UintegralTsProdOutMax=[]  UngainTsProdOutMin=[]  UngainTsProdOutMax=[]  IntegratorContinuousStateAttributes=''  IntegratorStateMustResolveToSignalObject=off  IntegratorRTWStateStorageClass=Auto  FilterContinuousStateAttributes=''  FilterStateMustResolveToSignalObject=off  FilterRTWStateStorageClass=Auto  ParallelPVariant=ExternalParameters  IdealPVariant=Disabled  IVariant=ExternalParameters  DVariant=Disabled  IntegratorVariant=Discrete  SatVariant=External  AWVariant=DiscClampingParallel  PCopyVariant=Disabled  TRVariant=Disabled  FdbkBlocksVariant=Forward  IdealPFdbkVariant=Disabled  SatFdbkVariant=Disabled  DerivativeFilterVariant=Disabled  NVariant=Disabled  NCopyVariant=Disabled_SignalSpec  FilterICVariant=Disabled  IntegratorICVariant=InternalICs  ExternalResetVariant=ExternalReset  TRSumVariant=Passthrough  SumFdbkVariant=Disabled  SumVariant=Sum_PI  TsampFilterVariant=InternalTs  TsampNgainVariant=Passthrough  TsampIntegralVariant=Passthrough  ExternalSaturationOutDataTypeStr=Inherit: Same as second input  aMode=0
  stab_roll_angle_rate_error_calc : Sum  Inputs=|+-
  roll_cc : Outport
  logging : Outport  Port=2
  wires:
  sys_input/1 -> Bus Selector/1
  Sum/1 -> roll_cc/1
  Mux/1 -> logging/1
  Bus Selector/1 -> Selector/1  "<gyro_radps>"
  Bus Selector/2 -> select_roll_PID/1  "<param>"
  select_roll_PID/1 -> Demux/1
  Demux/1 -> [PARAM_00]
  Demux/2 -> [PARAM_01]
  Demux/3 -> [PARAM_02]
  [PARAM_00] -> stab_roll_PID/2
  [PARAM_01] -> stab_roll_PID/3  "I_gain"
  [PARAM_02] -> Product/2  "D_gain"
  low_throttle_flag/1 -> stab_roll_PID/4
  Demux/4 -> [PARAM_10]
  [PARAM_15] -> Gain/1, stab_roll_PID/5
  Gain/1 -> stab_roll_PID/6
  Selector/1 -> roll_D_DLPF/1(raw_val), stab_roll_angle_rate_error_calc/2
  Demux/6 -> [PARAM_17]
  Discrete Derivative/1 -> Product/1
  [PARAM_17] -> roll_D_DLPF/2(freq_cut)
  roll_D_DLPF/1(filtered_val) -> Discrete Derivative/1
  [PARAM_10] -> Feed forward/1
  stab_roll_PID/1 -> Mux/2, Sum/2  "Roll_cmd"
  Feed forward/1 -> Sum/1
  Roll_rate_cmd_radps/1 -> Feed forward/2, stab_roll_angle_rate_error_calc/1, Mux/1
  stab_roll_angle_rate_error_calc/1 -> stab_roll_PID/1  "roll_angle_error"
  Product/1 -> Mux/3, Sum/3
  Demux/5 -> [PARAM_15]

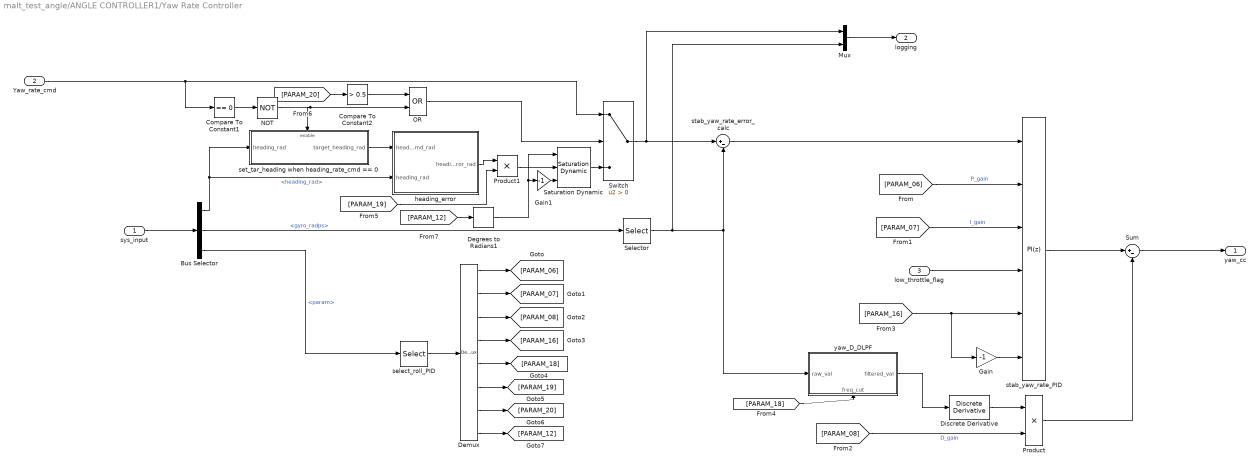
== system malt_test_angle/ANGLE CONTROLLER1/Yaw Rate Controller ==
  sys_input : Inport
  Yaw_rate_cmd : Inport  Port=2
  low_throttle_flag : Inport  Port=3
  Bus Selector : BusSelector  OutputSignals=Ins Data.heading_rad,Ins Data.gyro_radps,Telemetry Data.param
  Compare To Constant1 : simulink/Logic and Bit Operations/Compare To Constant  relop===  const=0  OutDataTypeStr=boolean
  Compare To Constant2 : simulink/Logic and Bit Operations/Compare To Constant  relop=>  const=0.5  OutDataTypeStr=boolean
  Degrees to Radians1 : simulink_extras/Transformations/Degrees to Radians
  Demux : Demux  Outputs=8
  Discrete Derivative : simulink/Quick Insert/Discrete/Discrete Derivative  gainval=1.0  ICPrevScaledInput=0.0  OutMin=[]  OutMax=[]  OutDataType=fixdt(1, 16)  OutScaling=2^-10  DoSatur=off
  Gain : Gain  Gain=-1
  Gain1 : Gain  Gain=-1
  Mux : Mux  Inputs=2
  NOT : Logic  Operator=NOT  IconShape=distinctive  AllPortsSameDT=off  OutDataTypeStr=boolean
  OR : Logic  Operator=OR  IconShape=distinctive  AllPortsSameDT=off  OutDataTypeStr=boolean
  Product : Product
  Product1 : Product
  Saturation Dynamic : simulink/Discontinuities/Saturation Dynamic  OutMin=[]  OutMax=[]  OutDataTypeStr=Inherit: Same as second input  OutDataType=fixdt(1, 16)  OutScaling=2^-10  DoSatur=off
  Selector : Selector  InputPortWidth=3  IndexOptions=Index vector (dialog)  Indices=3  OutputSizes=1
  Sum : Sum  Inputs=|+-
  Switch : Switch  Criteria=u2 > Threshold  SaturateOnIntegerOverflow=off  InputSameDT=off
  heading_error : Subsystem
  select_roll_PID : Selector  IndexMode=Zero-based  IndexOptions=Index vector (dialog)  Indices=[6 7 8 16 18 19 20 12]  OutputSizes=1
  set_tar_heading when heading_rate_cmd == 0 : Subsystem  TreatAsAtomicUnit=on
  stab_yaw_rate_PID : slpidlib/PID Controller  Controller=PI  Form=Parallel  TimeDomain=Discrete-time  UseExternalTs=off  SampleTime=framePeriod_s  IntegratorMethod=Forward Euler  FilterMethod=Forward Euler  ControllerParametersSource=external  P=1.85  I=0.01  UseKiTs=off  D=0  N=100  UseFilter=off  TunerSelectOption=Transfer Function Based (PID Tuner App)  InitialConditionSource=internal  InitialConditionForIntegrator=0  InitialConditionForFilter=0  DifferentiatorICPrevScaledInput=0  ExternalReset=either  TrackingMode=off  Kt=1  LimitOutput=on  SatLimitsSource=external  UpperSaturationLimit=inf  LowerSaturationLimit=-inf  LinearizeAsGain=off  AntiWindupMode=clamping  Kb=1  POutMin=[]  POutMax=[]  IOutMin=[]  IOutMax=[]  DOutMin=[]  DOutMax=[]  NOutMin=[]  NOutMax=[]  SumOutMin=[]  SumOutMax=[]  SaturationOutMin=[]  SaturationOutMax=[]  PParamMin=[]  PParamMax=[]  IParamMin=[]  IParamMax=[]  DParamMin=[]  DParamMax=[]  NParamMin=[]  NParamMax=[]  KbParamMin=[]  KbParamMax=[]  KtParamMin=[]  KtParamMax=[]  KbOutMin=[]  KbOutMax=[]  KtOutMin=[]  KtOutMax=[]  IntegratorOutMin=[]  IntegratorOutMax=[]  FilterOutMin=[]  FilterOutMax=[]  SumI1OutMin=[]  SumI1OutMax=[]  SumI2OutMin=[]  SumI2OutMax=[]  SumI3OutMin=[]  SumI3OutMax=[]  SumI4OutMin=[]  SumI4OutMax=[]  SumDOutMin=[]  SumDOutMax=[]  DifferentiatorOutMin=[]  DifferentiatorOutMax=[]  FilterDiffOutCoefMin=[]  FilterDiffOutCoefMax=[]  ReciprocalOutMin=[]  ReciprocalOutMax=[]  SumDenOutMin=[]  SumDenOutMax=[]  SumNumOutMin=[]  SumNumOutMax=[]  DivideOutMin=[]  DivideOutMax=[]  UdiffTsProdOutMin=[]  UdiffTsProdOutMax=[]  NTsProdOutMin=[]  NTsProdOutMax=[]  UintegralTsProdOutMin=[]  UintegralTsProdOutMax=[]  UngainTsProdOutMin=[]  UngainTsProdOutMax=[]  IntegratorContinuousStateAttributes=''  IntegratorStateMustResolveToSignalObject=off  IntegratorRTWStateStorageClass=Auto  FilterContinuousStateAttributes=''  FilterStateMustResolveToSignalObject=off  FilterRTWStateStorageClass=Auto  ParallelPVariant=ExternalParameters  IdealPVariant=Disabled  IVariant=ExternalParameters  DVariant=Disabled  IntegratorVariant=Discrete  SatVariant=External  AWVariant=DiscClampingParallel  PCopyVariant=Disabled  TRVariant=Disabled  FdbkBlocksVariant=Forward  IdealPFdbkVariant=Disabled  SatFdbkVariant=Disabled  DerivativeFilterVariant=Disabled  NVariant=Disabled  NCopyVariant=Disabled_SignalSpec  FilterICVariant=Disabled  IntegratorICVariant=InternalICs  ExternalResetVariant=ExternalReset  TRSumVariant=Passthrough  SumFdbkVariant=Disabled  SumVariant=Sum_PI  TsampFilterVariant=InternalTs  TsampNgainVariant=Passthrough  TsampIntegralVariant=Passthrough  ExternalSaturationOutDataTypeStr=Inherit: Same as second input  aMode=0
  stab_yaw_rate_error_calc : Sum  Inputs=|+-
  yaw_D_DLPF : Subsystem
      settings: PortSchema="{\"entries\":[{\"content\":{\"sides\":[{\"content\":{\"connectorIds\":[\"In1\"]},\"type\":\"ConnectorPlacement.EquallySpacedRectSide\",\"uuid\":\"20236834-aeb3-4c5b-bb2e-f84447e752b5\"},{\"content\":{\"connectorIds\":[\"Out1\"],\"side\":\"RIGHT\"},\"type\":\"ConnectorPlacement.EquallySpacedRectSide\",\"uuid\":\"d668f9a1-a3df-4207-8bf1-99fb838e59b2\"},{\"content\":{\"connectorIds\":[],\"side\":\"TOP\"},\"type\":\"ConnectorPlacement.EquallySpacedRectSide\",\"uuid\":\"66cceb06-f4bc-4278-b965-2427292e46df\"},{\"content\":{\"connectorIds\":[\"In2\"],\"side\":\"BOTTOM\"},\"type\":\"ConnectorPlacement.EquallySpacedRectSide\",\"uuid\":\"8171d125-c366-4676-8392-823b97a6c095\"}]},\"type\":\"ConnectorPlacement.EquallySpacedConnector\",\"uuid\":\"3dc29a9a-e794-478d-b7df-452e6c2d3f66\"}],\"packageUris\":[\"http://schema.mathworks.com/mf0/Connector/R2020b\"],\"version\":\"1.0\"}"
  yaw_cc : Outport
  logging : Outport  Port=2
  wires:
  sys_input/1 -> Bus Selector/1
  Bus Selector/2 -> Selector/1  "<gyro_radps>"
  Mux/1 -> logging/1
  stab_yaw_rate_PID/1 -> Sum/1
  Sum/1 -> yaw_cc/1
  Product/1 -> Sum/2
  Discrete Derivative/1 -> Product/1
  select_roll_PID/1 -> Demux/1
  Demux/1 -> [PARAM_06]
  Demux/3 -> [PARAM_08]
  Demux/2 -> [PARAM_07]
  Bus Selector/3 -> select_roll_PID/1  "<param>"
  [PARAM_06] -> stab_yaw_rate_PID/2  "P_gain"
  [PARAM_07] -> stab_yaw_rate_PID/3  "I_gain"
  [PARAM_08] -> Product/2  "D_gain"
  Selector/1 -> stab_yaw_rate_error_calc/2, yaw_D_DLPF/1(raw_val), Mux/2
  low_throttle_flag/1 -> stab_yaw_rate_PID/4
  Demux/4 -> [PARAM_16]
  [PARAM_16] -> Gain/1, stab_yaw_rate_PID/5
  Gain/1 -> stab_yaw_rate_PID/6
  Demux/5 -> [PARAM_18]
  Compare To Constant1/1 -> NOT/1
  NOT/1 -> OR/2, set_tar_heading when heading_rate_cmd == 0/Enable
  Bus Selector/1 -> set_tar_heading when heading_rate_cmd == 0/1(heading_rad), heading_error/2(heading_rad)  "<heading_rad>"
  Switch/1 -> Mux/1, stab_yaw_rate_error_calc/1
  Yaw_rate_cmd/1 -> Switch/1, Compare To Constant1/1
  Demux/6 -> [PARAM_19]
  Demux/7 -> [PARAM_20]
  heading_error/1(heading_error_rad) -> Product1/1
  [PARAM_19] -> Product1/2
  OR/1 -> Switch/2
  [PARAM_20] -> Compare To Constant2/1
  Compare To Constant2/1 -> OR/1
  set_tar_heading when heading_rate_cmd == 0/1(target_heading_rad) -> heading_error/1(heading_cmd_rad)
  Product1/1 -> Saturation Dynamic/2
  Saturation Dynamic/1 -> Switch/3
  Demux/8 -> [PARAM_12]
  [PARAM_12] -> Degrees to Radians1/1
  Gain1/1 -> Saturation Dynamic/3
  Degrees to Radians1/1 -> Saturation Dynamic/1, Gain1/1
  [PARAM_18] -> yaw_D_DLPF/2(freq_cut)
  yaw_D_DLPF/1(filtered_val) -> Discrete Derivative/1
  stab_yaw_rate_error_calc/1 -> stab_yaw_rate_PID/1

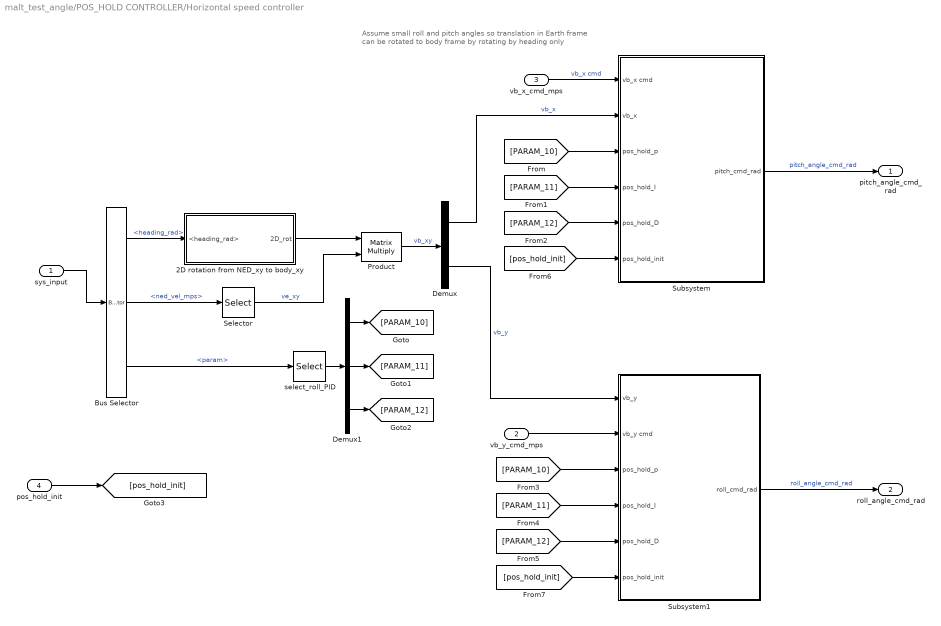
== system malt_test_angle/POS_HOLD CONTROLLER/Horizontal speed controller ==
  note: Assume small roll and pitch angles so translation in Earth frame can be rotated to body frame by rotating by heading only
  sys_input : Inport
  vb_y_cmd_mps : Inport  Port=2
  vb_x_cmd_mps : Inport  Port=3
  pos_hold_init : Inport  Port=4
  2D rotation from NED_xy to body_xy : Subsystem
  Bus Selector : BusSelector  OutputSignals=Navigation Filter Data.heading_rad,Navigation Filter Data.ned_vel_mps,Telemetry Data.param
  Demux : Demux  Outputs=2
  Demux1 : Demux  Outputs=3
  Product : Product  Multiplication=Matrix(*)
  Selector : Selector  InputPortWidth=3  IndexOptions=Index vector (dialog)  Indices=[1 2]  OutputSizes=1
  Subsystem : Subsystem
  Subsystem1 : Subsystem
  select_roll_PID : Selector  IndexMode=Zero-based  IndexOptions=Index vector (dialog)  Indices=[10 11 12]  OutputSizes=1
  pitch_angle_cmd_rad : Outport
  roll_angle_cmd_rad : Outport  Port=2
  wires:
  Subsystem1/1(roll_cmd_rad) -> roll_angle_cmd_rad/1  "roll_angle_cmd_rad"
  Subsystem/1(pitch_cmd_rad) -> pitch_angle_cmd_rad/1  "pitch_angle_cmd_rad"
  sys_input/1 -> Bus Selector/1
  Bus Selector/2 -> Selector/1  "<ned_vel_mps>"
  Selector/1 -> Product/2  "ve_xy"
  2D rotation from NED_xy to body_xy/1(2D_rot) -> Product/1
  Product/1 -> Demux/1  "vb_xy"
  Demux/2 -> Subsystem1/1(vb_y)  "vb_y"
  vb_x_cmd_mps/1 -> Subsystem/1(vb_x cmd)  "vb_x cmd"
  Demux/1 -> Subsystem/2(vb_x)  "vb_x"
  Bus Selector/1 -> 2D rotation from NED_xy to body_xy/1(<heading_rad>)  "<heading_rad>"
  vb_y_cmd_mps/1 -> Subsystem1/2(vb_y cmd)
  Demux1/3 -> [PARAM_12]
  Demux1/2 -> [PARAM_11]
  Demux1/1 -> [PARAM_10]
  select_roll_PID/1 -> Demux1/1
  Bus Selector/3 -> select_roll_PID/1  "<param>"
  [PARAM_10] -> Subsystem/3(pos_hold_p)
  [PARAM_11] -> Subsystem/4(pos_hold_I)
  [PARAM_12] -> Subsystem/5(pos_hold_D)
  [PARAM_10] -> Subsystem1/3(pos_hold_p)
  [PARAM_11] -> Subsystem1/4(pos_hold_I)
  [PARAM_12] -> Subsystem1/5(pos_hold_D)
  pos_hold_init/1 -> [pos_hold_init]
  [pos_hold_init] -> Subsystem/6(pos_hold_init)
  [pos_hold_init] -> Subsystem1/6(pos_hold_init)
